simulink model "test_function1"  (R2018a)
settings: Solver=VariableStepAuto  StartTime=0.0  StopTime=param_sim_time  RelTol=1e-3
values from neighbouring files (symbols this model uses):
  param_f = 0.001    [plot_task1.m]    (also in plot_test.m)
  param_g = 9.81    [plot_task1.m]    (also in plot_test.m)
  param_k1 = 10800    [plot_task1.m]    (also in plot_test.m)
  param_m1 = 0.25    [plot_task1.m]    (also in plot_test.m)
  param_N = 8    [plot_task1.m]    (also in plot_test.m)
  param_v = 2500    [plot_task1.m]    (also in plot_test.m)
  param_y2 = (-param_g * (param_m1 + param_m2)) / param_k2    (= -0.000113541666667)    [plot_task1.m]    (also in plot_test.m = -0.0001135)
  param_ys0 = 0.022    [plot_task1.m]    (also in plot_test.m = 0.09)
  params = struct    [Parameter_t1.m]    (also in sDE_dispIn.m = block.DialogPrm(1).Data)
settings Model: Creator=Matthias  LastModifiedBy=Matthias

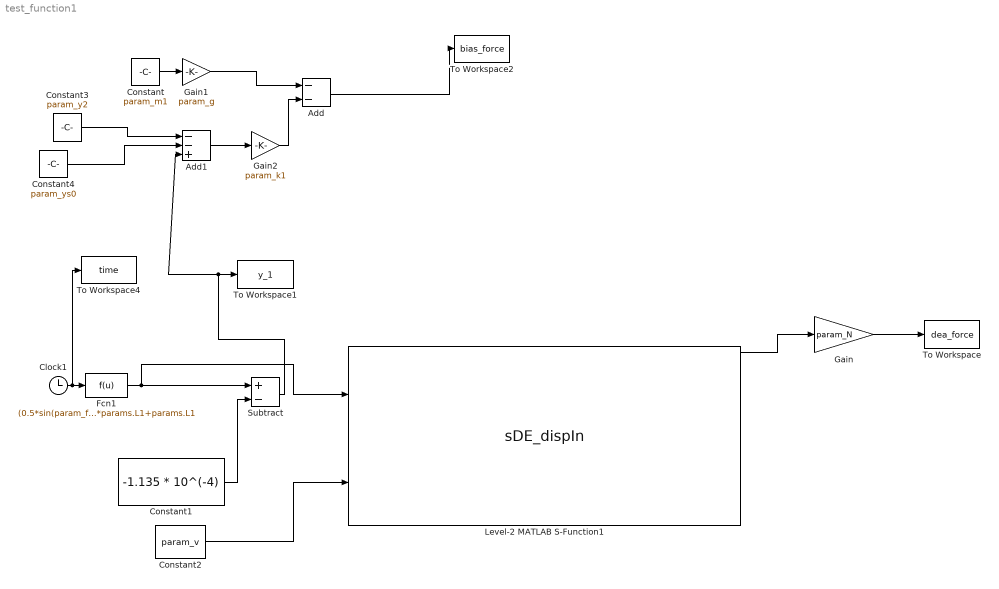
== system test_function1 ==
  Add : Sum  Inputs=--
  Add1 : Sum  Inputs=--+
  Clock1 : Clock
  Constant : Constant  Value=param_m1
  Constant1 : Constant  Value=-1.135 * 10^(-4)
  Constant2 : Constant  Value=param_v
  Constant3 : Constant  Value=param_y2
  Constant4 : Constant  Value=param_ys0
  Fcn1 : Fcn  Expr=(0.5*sin(param_f*u)+0.5)*params.L1+params.L1
  Gain : Gain  Gain=param_N
  Gain1 : Gain  Gain=param_g
  Gain2 : Gain  Gain=param_k1
  Level-2 MATLAB S-Function1 : M-S-Function  FunctionName=sDE_dispIn  Parameters=params, initConds
      mask Display:
      | color('black');
      | patch(4*[-1 1 1 -1],1.75*[-1 -1 1 1],[1 1 1]);
      | patch(2*[-1 1 1 -1],1.2*[-1 -1 1 1],[0 0 0]);
      | patch(1.95*[-1 1 1 -1],0.8*[-1 -1 1 1],[1 1 1]);
      | disp('DE Actuator');
      | 
      | color('blue');
      | port_label('input', 1, 'l_1 [m]','texmode','on');
      | port_label('input', 2, 'v [V]','texmode','on');
      | 
      | color('red');
      | port_label('output', 1, 'F_1 [N]','texmode','on');
      | port_label('output', 2, 'x_{v1} [-]','texmode','on');
      | port_label('output', 3, 'x_{v2} [-]','texmode','on');
      | port_label('output', 4, '\epsilon_2 [-]','texmode','on');
      | port_label('output', 5, 'q [C]','texmode','on');
      | port_label('output', 6, '\epsilon_1 [-]','texmode','on');
      | port_label('output', 7, '\sigma_1 [Pa]','texmode','on');
      | port_label('output', 8, 'i [A]','texmode','on');
      | port_label('output', 9, 'v_{DE} [V]','texmode','on');
      | port_label('output', 10, 'C [F]','texmode','on');
  Subtract : Sum  Inputs=+-
  To Workspace : ToWorkspace  VariableName=dea_force  SampleTime=-1
  To Workspace1 : ToWorkspace  VariableName=y_1  SampleTime=-1
  To Workspace2 : ToWorkspace  VariableName=bias_force  SampleTime=-1
  To Workspace4 : ToWorkspace  VariableName=time  SampleTime=-1
  wires:
  Constant1/1 -> Subtract/2
  Constant2/1 -> Level-2 MATLAB S-Function1/2
  Gain/1 -> To Workspace/1
  Level-2 MATLAB S-Function1/1 -> Gain/1
  Clock1/1 -> To Workspace4/1, Fcn1/1
  Fcn1/1 -> Level-2 MATLAB S-Function1/1, Subtract/1
  Constant/1 -> Gain1/1
  Gain1/1 -> Add/1
  Constant3/1 -> Add1/1
  Constant4/1 -> Add1/2
  Subtract/1 -> Add1/3, To Workspace1/1
  Add1/1 -> Gain2/1
  Gain2/1 -> Add/2
  Add/1 -> To Workspace2/1
